simulink model "sampleModel1802_2_sub_sub"  (R2023a)
settings: Solver=VariableStepAuto  StartTime=0.0  StopTime=10.0  RelTol=1e-3
libraries: hdlsllib x3, simulink x1
settings Model: Creator=user1  LastModifiedBy=user1

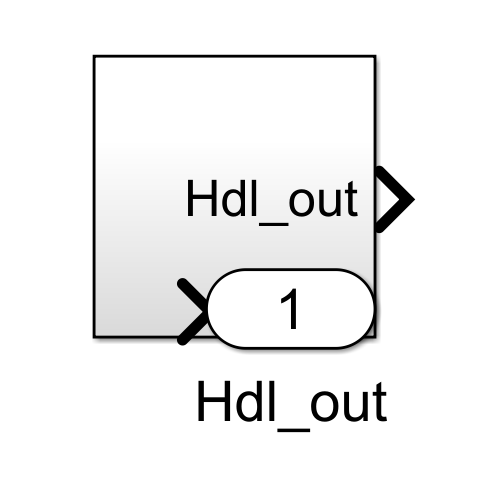
[thumbnail: Simulink's stored preview of the top-level diagram]
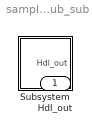
== system sampleModel1802_2_sub_sub ==
  Subsystem : Subsystem
  Hdl_out : Outport  OutDataTypeStr=uint8

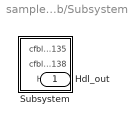
== system sampleModel1802_2_sub_sub/Subsystem ==
  Subsystem : Subsystem
  Hdl_out : Outport  OutDataTypeStr=uint8

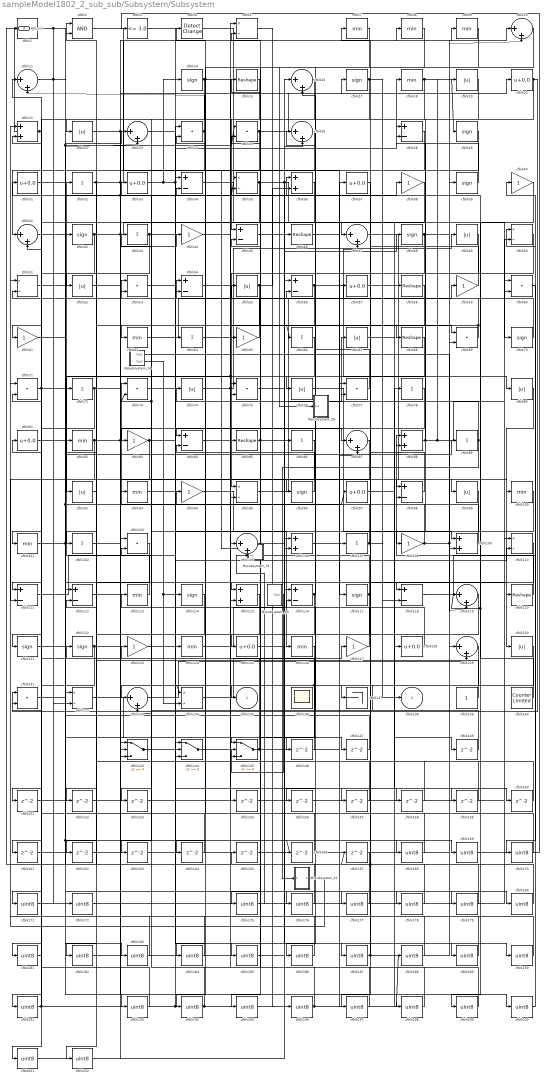
== system sampleModel1802_2_sub_sub/Subsystem/Subsystem ==
  Mysubsystem_14 : Subsystem  TreatAsAtomicUnit=on  RTWFcnName=Mysubsystem_14
      settings: RTWFcnNameOpts=User specified  RTWFileNameOpts=Use function name
  Mysubsystem_28 : Subsystem  TreatAsAtomicUnit=on  RTWFcnName=Mysubsystem_28
      settings: RTWFcnNameOpts=User specified  RTWFileNameOpts=Use function name
  Mysubsystem_31 : Subsystem  TreatAsAtomicUnit=on  RTWFcnName=Mysubsystem_31
      settings: RTWFcnNameOpts=User specified  RTWFileNameOpts=Use function name
  Mysubsystem_41 : Subsystem  TreatAsAtomicUnit=on  RTWFcnName=Mysubsystem_41
      settings: RTWFcnNameOpts=User specified  RTWFileNameOpts=Use function name
  Mysubsystem_49 : Subsystem  TreatAsAtomicUnit=on  RTWFcnName=Mysubsystem_49
      settings: RTWFcnNameOpts=User specified  RTWFileNameOpts=Use function name
  cfblk1 : hdlsllib/Logic and Bit Operations/Compare To Zero  relop=<=  OutDataTypeStr=uint8
  cfblk{10..11,16,23,26,41,47,87,105,119,129,133} (12 alike) : Sum  Inputs=|++  OutDataTypeStr=uint8
  cfblk{7..9,18,63,82,93,100..101,113,124,126} (12 alike) : MinMax  OutDataTypeStr=uint8
  cfblk{32,43,64,66,72,78,86,89,102,107} (10 alike) : Sum  Inputs=+  OutDataTypeStr=uint8
  cfblk{24..25,53,60,69,71,73,75,77,103,131} (11 alike) : DotProduct  OutDataTypeStr=uint8
  cfblk{21,36,88,106,109,115} (6 alike) : Sum  OutDataTypeStr=uint8
  cfblk{38,40,44,59,61,65,83,94,108,123,127} (11 alike) : Gain  OutDataTypeStr=uint8
  cfblk{5,35,50..51,95,110,132,134} (8 alike) : Product  Inputs=*/  OutDataTypeStr=uint8  RndMeth=Zero  SaturateOnIntegerOverflow=on
  cfblk{28,34,45,54,56,84,98,111..112,116,118} (11 alike) : Sum  Inputs=+-  OutDataTypeStr=uint8
  cfblk{14,17,29,39,42,48,70,96,114,117,121..122} (12 alike) : Signum
  cfblk{15,46,58,68,85,120} (6 alike) : Reshape
  cfblk{20,31,33,37,57,81,97,125,128} (9 alike) : Bias  Bias=0.0  SaturateOnIntegerOverflow=off
  cfblk{19,22,49,52,55,67,74,76,80,92,99,130} (12 alike) : Abs  OutDataTypeStr=uint8  SaturateOnIntegerOverflow=off
  cfblk136 : Scope
      settings: Floating=on
  cfblk137 : Terminator
  cfblk139 : Constant  OutDataTypeStr=uint8  SampleTime=-1
  cfblk140 : hdlsllib/Sources/Counter Limited  uplimit=7  tsamp=-1
  cfblk143 : Switch  OutDataTypeStr=uint8  SaturateOnIntegerOverflow=off  InputSameDT=off
  cfblk144 : Switch  OutDataTypeStr=uint8  SaturateOnIntegerOverflow=off  InputSameDT=off
  cfblk145 : Switch  OutDataTypeStr=uint8  SaturateOnIntegerOverflow=off  InputSameDT=off
  cfblk{146..147,149,151..153,155..167} (19 alike) : Delay  SampleTime=1
  cfblk{168..172,175..191,193..202} (32 alike) : DataTypeConversion  OutDataTypeStr=uint8  SaturateOnIntegerOverflow=off  RndMeth=Floor
  cfblk2 : Logic  AllPortsSameDT=off  OutDataTypeStr=boolean
  cfblk3 : hdlsllib/Logic and Bit Operations/Compare To Constant  relop=<=  const=3.0  OutDataTypeStr=uint8
  cfblk4 : simulink/Logic and Bit Operations/Detect Change  vinit=0  OutDataTypeStr=uint8
      settings: LibrarySourceBlock=|
      | hdlsllib/Logic and Bit
      | Operations/Detect
      | Change
  cfblk135 : Outport  OutDataTypeStr=uint8  VectorParamsAs1DForOutWhenUnconnected=off
  cfblk138 : Outport  Port=2  OutDataTypeStr=uint8  VectorParamsAs1DForOutWhenUnconnected=off
  Hdl_out : Outport  Port=3  OutDataTypeStr=uint8
  wires:
  Mysubsystem_49/1(Out1) -> cfblk145/2
  Mysubsystem_41/1(Out1) -> cfblk21/1
  cfblk175/1 -> Mysubsystem_31/2(In2)
  cfblk26/1 -> Mysubsystem_31/1(In1)
  cfblk9/1 -> Mysubsystem_28/1(In1)
  Mysubsystem_14/1(Out1) -> cfblk109/2
  Mysubsystem_14/2(Out2) -> cfblk114/1, cfblk134/2
  cfblk202/1 -> cfblk86/1
  cfblk114/1 -> cfblk202/1
  cfblk201/1 -> cfblk143/1
  cfblk86/1 -> cfblk201/1
  cfblk200/1 -> cfblk40/1
  cfblk199/1 -> cfblk106/1
  cfblk40/1 -> cfblk199/1
  cfblk198/1 -> cfblk5/2
  cfblk152/1 -> cfblk198/1
  cfblk197/1 -> cfblk5/1
  cfblk110/1 -> cfblk197/1
  cfblk196/1 -> cfblk73/2, cfblk43/1, cfblk87/2
  cfblk195/1 -> cfblk78/1
  cfblk7/1 -> cfblk195/1
  cfblk194/1 -> cfblk37/1, cfblk33/1
  cfblk193/1 -> cfblk21/2
  cfblk191/1 -> cfblk188/1, cfblk144/3, cfblk71/2
  cfblk190/1 -> cfblk165/1
  cfblk105/1 -> cfblk190/1
  cfblk189/1 -> cfblk71/1
  cfblk165/1 -> cfblk189/1
  cfblk188/1 -> cfblk93/1
  cfblk187/1 -> cfblk167/1, cfblk77/2, cfblk39/1
  cfblk186/1 -> cfblk123/1
  cfblk119/1 -> cfblk186/1
  cfblk185/1 -> cfblk46/1
  cfblk123/1 -> cfblk185/1
  cfblk184/1 -> cfblk103/2
  cfblk183/1 -> cfblk103/1
  cfblk182/1 -> cfblk116/1
  cfblk103/1 -> cfblk182/1
  cfblk181/1 -> cfblk51/2
  cfblk180/1 -> cfblk51/1
  cfblk163/1 -> cfblk180/1
  cfblk179/1 -> cfblk24/1
  cfblk51/1 -> cfblk179/1
  cfblk178/1 -> cfblk112/2
  cfblk23/1 -> cfblk178/1
  cfblk177/1 -> cfblk112/1
  cfblk155/1 -> cfblk177/1
  cfblk176/1 -> cfblk25/2
  cfblk112/1 -> cfblk176/1
  cfblk172/1 -> cfblk60/2
  cfblk171/1 -> cfblk60/1
  cfblk170/1 -> cfblk94/1
  cfblk60/1 -> cfblk170/1
  cfblk169/1 -> cfblk3/1
  cfblk168/1 -> cfblk55/1
  cfblk3/1 -> cfblk168/1
  cfblk167/1 -> cfblk1/1
  cfblk166/1 -> cfblk24/2
  cfblk164/1 -> cfblk131/2
  cfblk162/1 -> cfblk34/1
  cfblk115/1 -> cfblk162/1
  cfblk161/1 -> cfblk69/2
  cfblk160/1 -> cfblk2/2
  cfblk67/1 -> cfblk160/1
  cfblk159/1 -> cfblk45/2
  cfblk53/1 -> cfblk159/1
  cfblk158/1 -> cfblk144/1
  cfblk157/1 -> cfblk133/2
  cfblk84/1 -> cfblk157/1
  cfblk156/1 -> cfblk129/1
  cfblk99/1 -> cfblk156/1
  cfblk44/1 -> cfblk155/1
  cfblk153/1 -> cfblk110/1
  cfblk36/1 -> cfblk153/1
  cfblk151/1 -> cfblk16/1
  cfblk149/1 -> cfblk116/2
  cfblk97/1 -> cfblk149/1
  cfblk147/1 -> cfblk132/1
  cfblk41/1 -> cfblk147/1
  cfblk146/1 -> cfblk11/1
  cfblk58/1 -> cfblk146/1
  cfblk38/1 -> cfblk72/1
  cfblk48/1 -> cfblk10/1, cfblk96/1
  cfblk46/1 -> cfblk77/1
  cfblk116/1 -> cfblk16/2, cfblk125/1
  cfblk19/1 -> cfblk108/1
  cfblk121/1 -> cfblk97/1, cfblk23/2
  cfblk130/1 -> cfblk143/2
  cfblk34/1 -> cfblk128/1
  cfblk39/1 -> cfblk18/1
  cfblk65/1 -> cfblk42/1
  cfblk1/1 -> cfblk172/1, cfblk193/1
  cfblk100/1 -> cfblk133/1
  cfblk83/1 -> cfblk106/2, cfblk143/3
  cfblk28/1 -> cfblk61/1
  cfblk52/1 -> cfblk100/1
  cfblk24/1 -> cfblk11/2, cfblk63/1
  cfblk76/1 -> cfblk109/1
  cfblk82/1 -> cfblk53/2, cfblk145/3, cfblk111/2
  cfblk96/1 -> cfblk84/2
  cfblk144/1 -> cfblk88/2
  cfblk69/1 -> cfblk41/2, cfblk66/1
  cfblk125/1 -> cfblk48/1
  cfblk2/1 -> cfblk117/1
  cfblk108/1 -> cfblk119/2, cfblk10/2, cfblk98/2
  cfblk8/1 -> cfblk84/1
  cfblk59/1 -> cfblk34/2
  cfblk131/1 -> cfblk89/1
  cfblk122/1 -> cfblk17/1, cfblk171/1
  cfblk57/1 -> cfblk58/1
  cfblk132/1 -> cfblk145/1
  cfblk95/1 -> cfblk67/1
  cfblk133/1 -> cfblk129/2
  cfblk55/1 -> cfblk36/2, cfblk152/1
  cfblk89/1 -> Mysubsystem_41/1(In1), cfblk4/1
  cfblk117/1 -> cfblk74/1, cfblk184/1
  cfblk18/1 -> cfblk29/1, cfblk105/2
  cfblk143/1 -> cfblk110/2
  cfblk73/1 -> cfblk124/1
  cfblk124/1 -> cfblk26/2
  cfblk77/1 -> cfblk26/1
  cfblk49/1 -> cfblk95/2
  cfblk43/1 -> cfblk151/1, cfblk169/1
  cfblk101/1 -> cfblk115/1, cfblk35/2
  cfblk54/1 -> cfblk120/1
  cfblk75/1 -> cfblk38/1
  cfblk25/1 -> cfblk20/1, cfblk54/2
  cfblk106/1 -> cfblk57/1
  cfblk72/1 -> cfblk8/1, cfblk35/1, cfblk161/1
  cfblk45/1 -> cfblk69/1
  cfblk120/1 -> cfblk88/1
  cfblk14/1 -> cfblk68/1, cfblk164/1, cfblk83/1
  cfblk139/1 -> cfblk82/1
  cfblk93/1 -> cfblk187/1
  cfblk111/1 -> cfblk64/1
  cfblk134/1 -> cfblk127/1
  cfblk31/1 -> cfblk25/1, cfblk23/1
  cfblk128/1 -> cfblk113/1
  cfblk88/1 -> cfblk50/2, cfblk19/1, cfblk28/2
  cfblk107/1 -> cfblk15/1, cfblk138/1
  cfblk35/1 -> cfblk70/1, cfblk158/1, cfblk111/1
  cfblk63/1 -> cfblk47/2
  cfblk127/1 -> cfblk54/1
  cfblk140/1 -> cfblk119/1, cfblk31/1
  cfblk29/1 -> cfblk41/1
  cfblk16/1 -> cfblk85/1
  cfblk145/1 -> cfblk107/1, cfblk81/1
  cfblk94/1 -> cfblk126/1
  cfblk70/1 -> cfblk53/1
  cfblk92/1 -> cfblk2/1
  cfblk61/1 -> cfblk75/1
  cfblk20/1 -> cfblk131/1, cfblk22/1
  cfblk102/1 -> cfblk44/1
  cfblk11/1 -> cfblk132/2, cfblk200/1
  cfblk47/1 -> cfblk99/1
  cfblk109/1 -> cfblk73/1
  cfblk22/1 -> cfblk105/1, cfblk87/1
  cfblk50/1 -> cfblk65/1
  cfblk21/1 -> cfblk191/1, Hdl_out/1
  cfblk80/1 -> cfblk130/1
  cfblk81/1 -> cfblk166/1, cfblk183/1
  cfblk10/1 -> cfblk76/1
  cfblk87/1 -> cfblk102/1
  cfblk4/1 -> cfblk56/1
  cfblk126/1 -> cfblk134/1, cfblk175/1
  cfblk64/1 -> cfblk95/1
  cfblk17/1 -> cfblk121/1, cfblk118/2
  cfblk129/1 -> cfblk122/1
  cfblk56/1 -> cfblk80/1, cfblk144/2
  cfblk5/1 -> cfblk196/1
  cfblk15/1 -> cfblk45/1
  cfblk118/1 -> cfblk50/1
  cfblk74/1 -> cfblk49/1, cfblk56/2
  cfblk78/1 -> cfblk194/1
  cfblk71/1 -> cfblk36/1, cfblk181/1
  cfblk68/1 -> cfblk115/2, cfblk163/1
  cfblk98/1 -> cfblk7/1
  cfblk37/1 -> cfblk137/1
  cfblk66/1 -> cfblk92/1
  cfblk32/1 -> cfblk9/1, cfblk98/1, cfblk52/1
  cfblk85/1 -> cfblk59/1, cfblk135/1
  cfblk113/1 -> cfblk32/1
  cfblk33/1 -> cfblk118/1, cfblk28/1, cfblk14/1
  cfblk42/1 -> cfblk47/1, cfblk75/2, cfblk101/1

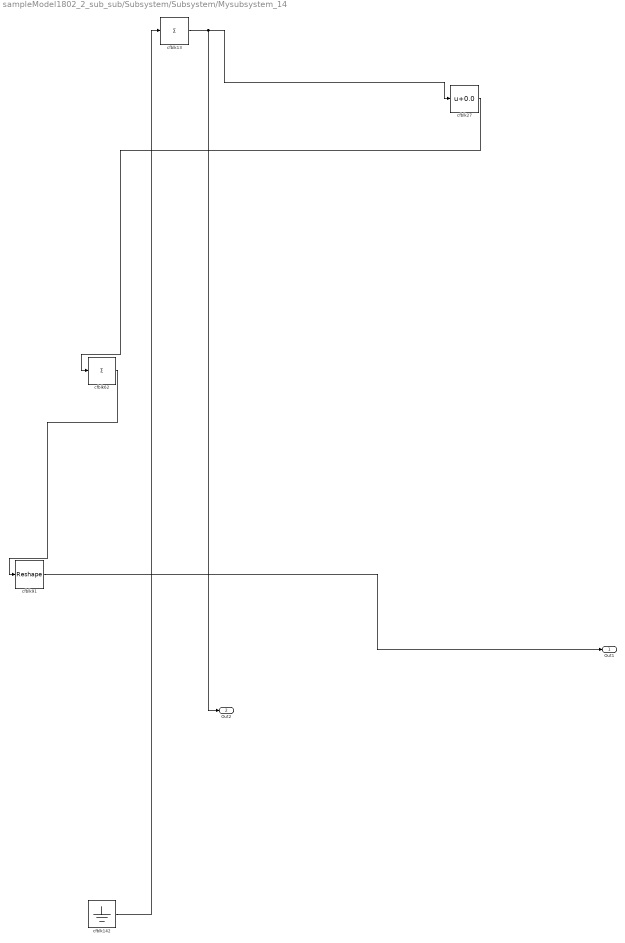
== system sampleModel1802_2_sub_sub/Subsystem/Subsystem/Mysubsystem_14 ==
  cfblk13 : Sum  Inputs=+
  cfblk142 : Ground
  cfblk27 : Bias  Bias=0.0  SaturateOnIntegerOverflow=off
  cfblk62 : Sum  Inputs=+
  cfblk91 : Reshape
  Out1 : Outport
  Out2 : Outport  Port=2
  wires:
  cfblk142/1 -> cfblk13/1
  cfblk27/1 -> cfblk62/1
  cfblk91/1 -> Out1/1
  cfblk13/1 -> Out2/1, cfblk27/1
  cfblk62/1 -> cfblk91/1

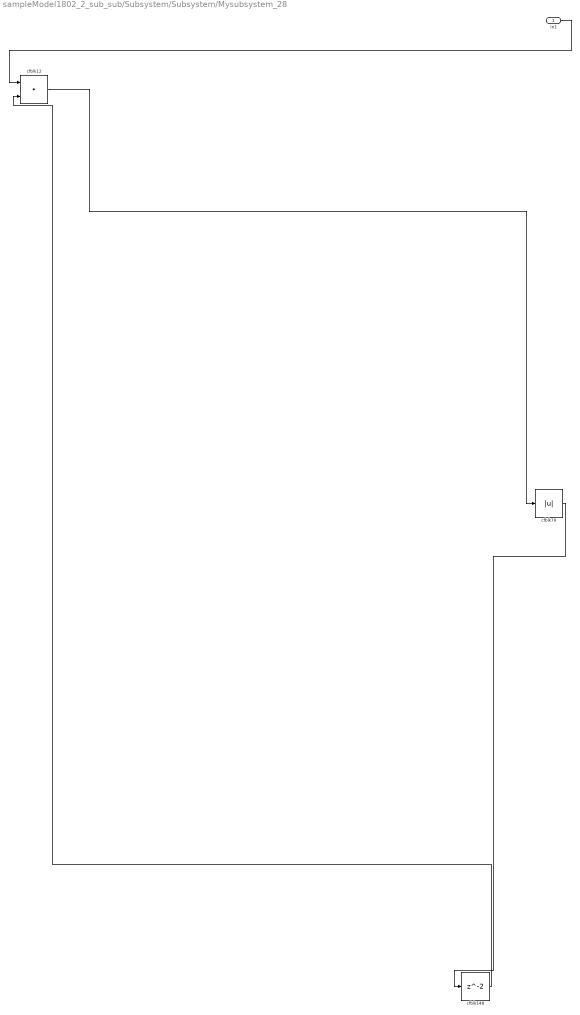
== system sampleModel1802_2_sub_sub/Subsystem/Subsystem/Mysubsystem_28 ==
  In1 : Inport
  cfblk12 : DotProduct  OutDataTypeStr=Inherit: Inherit via internal rule
  cfblk148 : Delay  SampleTime=1
  cfblk79 : Abs  SaturateOnIntegerOverflow=off
  wires:
  cfblk79/1 -> cfblk148/1
  cfblk12/1 -> cfblk79/1
  cfblk148/1 -> cfblk12/2
  In1/1 -> cfblk12/1

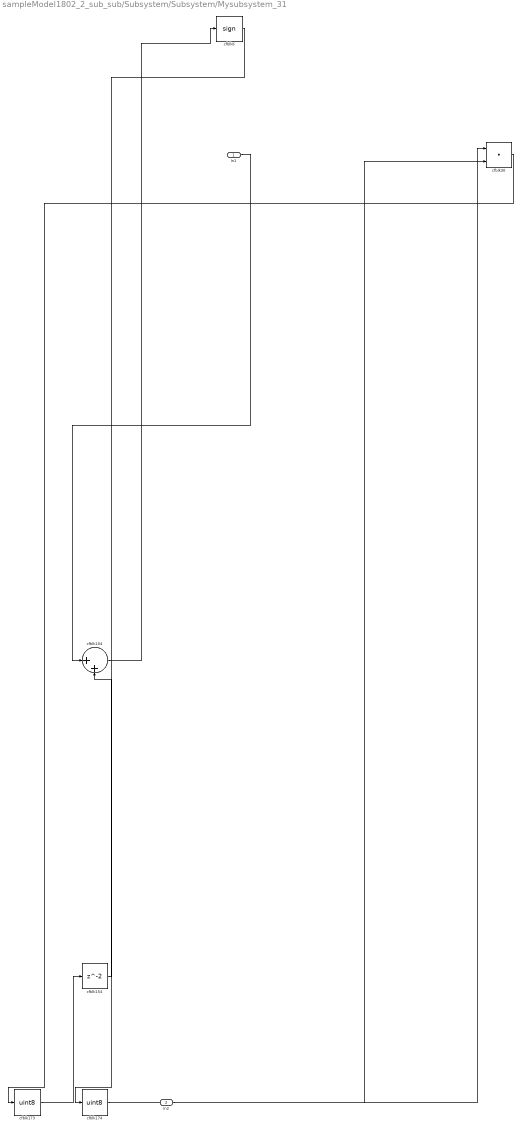
== system sampleModel1802_2_sub_sub/Subsystem/Subsystem/Mysubsystem_31 ==
  In1 : Inport
  In2 : Inport  Port=2
  cfblk104 : Sum  Inputs=|++
  cfblk154 : Delay  SampleTime=1
  cfblk173 : DataTypeConversion  OutDataTypeStr=uint8  SaturateOnIntegerOverflow=off  RndMeth=Floor
  cfblk174 : DataTypeConversion  OutDataTypeStr=uint8  SaturateOnIntegerOverflow=off  RndMeth=Floor
  cfblk30 : DotProduct  OutDataTypeStr=Inherit: Inherit via internal rule
  cfblk6 : Signum
  wires:
  In2/1 -> cfblk30/2
  cfblk104/1 -> cfblk6/1
  cfblk30/1 -> cfblk173/1
  cfblk154/1 -> cfblk104/2
  cfblk173/1 -> cfblk154/1
  cfblk6/1 -> cfblk174/1
  cfblk174/1 -> cfblk30/1
  In1/1 -> cfblk104/1

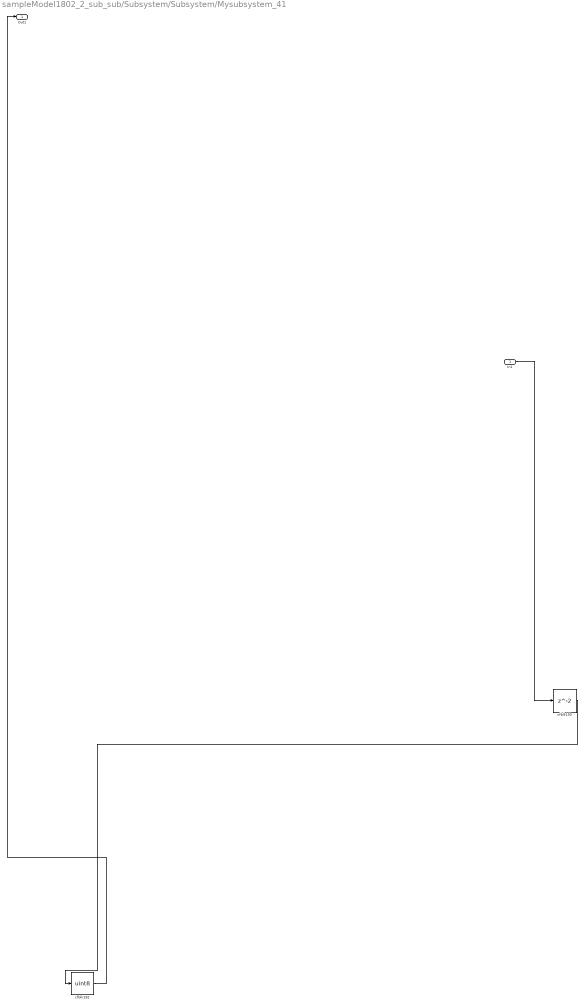
== system sampleModel1802_2_sub_sub/Subsystem/Subsystem/Mysubsystem_41 ==
  In1 : Inport
  cfblk150 : Delay  SampleTime=1
  cfblk192 : DataTypeConversion  OutDataTypeStr=uint8  SaturateOnIntegerOverflow=off  RndMeth=Floor
  Out1 : Outport
  wires:
  cfblk150/1 -> cfblk192/1
  In1/1 -> cfblk150/1
  cfblk192/1 -> Out1/1

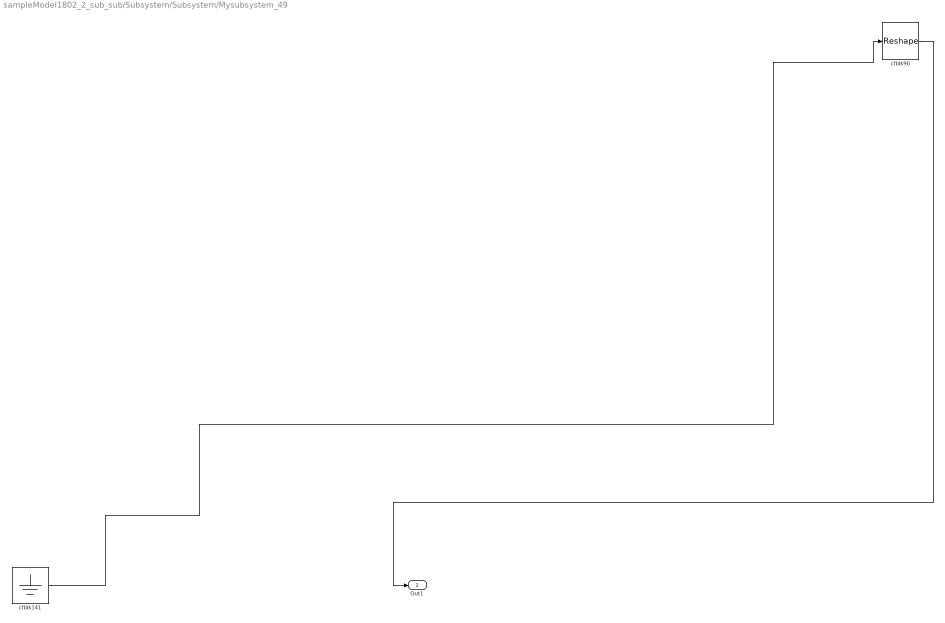
== system sampleModel1802_2_sub_sub/Subsystem/Subsystem/Mysubsystem_49 ==
  cfblk141 : Ground
  cfblk90 : Reshape
  Out1 : Outport
  wires:
  cfblk141/1 -> cfblk90/1
  cfblk90/1 -> Out1/1
